simulink model "lab3_5_1"  (R2018a)
settings: Solver=VariableStepAuto  StartTime=0.0  StopTime=1500*Ts  RelTol=1e-3
values from neighbouring files (symbols this model uses):
  scramblerLocal = [3 5]    [lab3.m]
  scramblerRemote = [5 7]    [lab3.m]
  Ts = 1    [lab3.m]
settings Model: Creator=leonardopedroso  LastModifiedBy=leonardopedroso

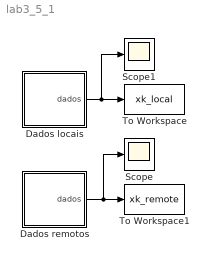
== system lab3_5_1 ==
  Dados locais : Subsystem
  Dados remotos : Subsystem
  Scope : Scope
  Scope1 : Scope
  To Workspace : ToWorkspace  VariableName=xk_local  SaveFormat=Timeseries  SampleTime=Ts/10
  To Workspace1 : ToWorkspace  VariableName=xk_remote  SaveFormat=Timeseries  SampleTime=Ts/10
  wires:
  Dados remotos/1(dados) -> Scope/1, To Workspace1/1
  Dados locais/1(dados) -> Scope1/1, To Workspace/1

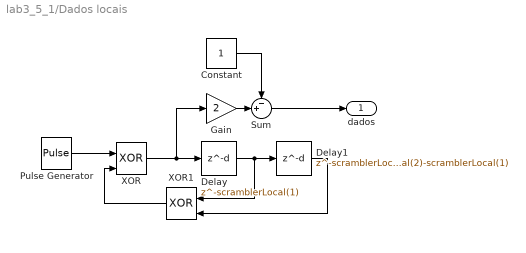
== system lab3_5_1/Dados locais ==
  Constant : Constant
  Delay : Delay  DelayLength=scramblerLocal(1)  SampleTime=Ts
  Delay1 : Delay  DelayLength=scramblerLocal(2)-scramblerLocal(1)  SampleTime=Ts
  Gain : Gain  Gain=2
  Pulse Generator : DiscretePulseGenerator  PulseType=Time based  Period=2*Ts  PulseWidth=50
  Sum : Sum  Inputs=-+|
  XOR : Logic  Operator=XOR  IconShape=distinctive  AllPortsSameDT=off  OutDataTypeStr=boolean
  XOR1 : Logic  Operator=XOR  IconShape=distinctive  AllPortsSameDT=off  OutDataTypeStr=boolean
  dados : Outport
  wires:
  Pulse Generator/1 -> XOR/1
  XOR1/1 -> XOR/2
  Delay/1 -> XOR1/1, Delay1/1
  Delay1/1 -> XOR1/2
  Gain/1 -> Sum/2
  Constant/1 -> Sum/1
  XOR/1 -> Delay/1, Gain/1
  Sum/1 -> dados/1

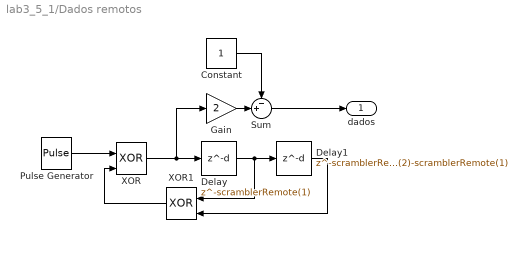
== system lab3_5_1/Dados remotos ==
  Constant : Constant
  Delay : Delay  DelayLength=scramblerRemote(1)  SampleTime=Ts
  Delay1 : Delay  DelayLength=scramblerRemote(2)-scramblerRemote(1)  SampleTime=Ts
  Gain : Gain  Gain=2
  Pulse Generator : DiscretePulseGenerator  PulseType=Time based  Period=2*Ts  PulseWidth=50
  Sum : Sum  Inputs=-+|
  XOR : Logic  Operator=XOR  IconShape=distinctive  AllPortsSameDT=off  OutDataTypeStr=boolean
  XOR1 : Logic  Operator=XOR  IconShape=distinctive  AllPortsSameDT=off  OutDataTypeStr=boolean
  dados : Outport
  wires:
  Pulse Generator/1 -> XOR/1
  XOR1/1 -> XOR/2
  Delay/1 -> XOR1/1, Delay1/1
  Delay1/1 -> XOR1/2
  Gain/1 -> Sum/2
  Constant/1 -> Sum/1
  XOR/1 -> Delay/1, Gain/1
  Sum/1 -> dados/1
